simulink model "Tank1"  (R2015a)
settings: Solver=ode45  StartTime=0.0  StopTime=1000  RelTol=1e-3
undefined symbols (not defined in the file): b
libraries: TTLibrary x2
settings Model: CovSFcnEnable=off  Creator=blindner  LastModifiedBy=blindner
settings DataIOCC: ExternalInput=getinputstruct(Tank1OPTrimmed)  InitialState=getstatestruct(Tank1OPTrimmed)  SaveOutput=off  SaveTime=off
settings DebuggingCC: SolverPrmCheckMsg=warning

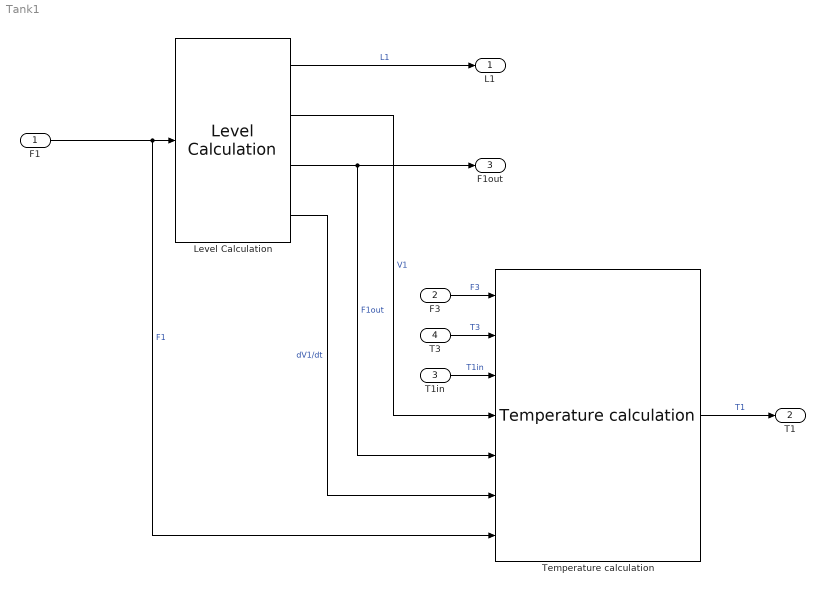
== system Tank1 ==
  F1 : Inport  OutDataTypeStr=double  PortDimensions=1  SampleTime=0
  F3 : Inport  Port=2  OutDataTypeStr=double  PortDimensions=1  SampleTime=0
  T1in : Inport  Port=3  OutDataTypeStr=double  PortDimensions=1  SampleTime=0
  T3 : Inport  Port=4  OutDataTypeStr=double  PortDimensions=1  SampleTime=0
  Level Calculation : TTLibrary/Level Calculation  kl=kl  Area=Area  Li=L1i  numIn=1
  Temperature calculation : TTLibrary/Temperature calculation  Ti=T1i  p=p  cp=cp  b=b  aHeat=aHeat  numIn=1
  L1 : Outport  OutDataTypeStr=double  PortDimensions=1  SampleTime=0
  "T1 " : Outport  Port=2  OutDataTypeStr=double  PortDimensions=1  SampleTime=0
  F1out : Outport  Port=3  OutDataTypeStr=double  PortDimensions=1  SampleTime=0
  wires:
  T1in/1 -> Temperature calculation/3  "T1in"
  T3/1 -> Temperature calculation/2  "T3"
  Level Calculation/1 -> L1/1  "L1"
  Level Calculation/3 -> F1out/1, Temperature calculation/5  "F1out"
  F3/1 -> Temperature calculation/1  "F3"
  F1/1 -> Level Calculation/1, Temperature calculation/7  "F1"
  Temperature calculation/1 -> "T1 "/1  "T1"
  Level Calculation/4 -> Temperature calculation/6  "dV1/dt"
  Level Calculation/2 -> Temperature calculation/4  "V1"
